simulink model "buckboostSMC2"  (R2024a)
settings: Solver=ode2  StartTime=0.0  StopTime=20  FixedStep=0.0001  RelTol=1e-3
InitFcn:
  | paramsTCST
values from neighbouring files (symbols this model uses):
  C = 2610*10^-6    (= 0.00261)    [SITLparameters.m]
  k1 = 0.022    [SITLparameters.m]
  k2 = 10    [SITLparameters.m]
  L = 2010*10^-6    (= 0.00201)    [SITLparameters.m]
  R = 25    [SITLparameters.m]
undefined symbols (not defined in the file or in its folder): gains, Lsig, Msig, params, Vd, x2d
settings Model: Creator=gerar  LastModifiedBy=rodol
settings ModelReferenceCC: EnableRefExpFcnMdlSchedulingChecks=on
settings RTWCC: GPUComputeCapability=3.5

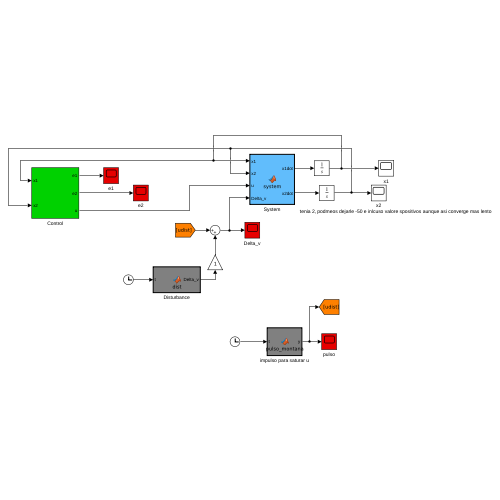
[thumbnail: Simulink's stored preview of the top-level diagram]
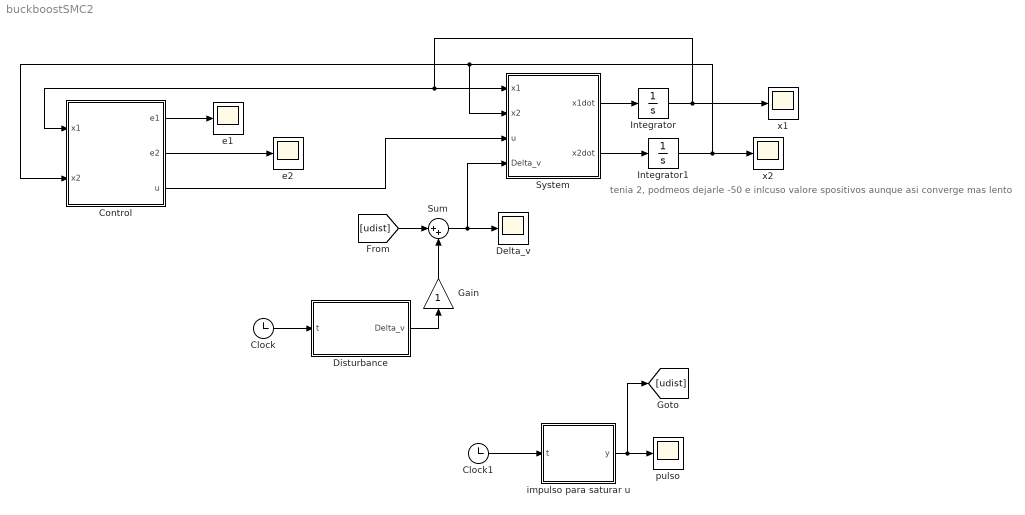
== system buckboostSMC2 ==
  note: tenia 2, podmeos dejarle -50 e inlcuso valore spositivos aunque asi converge mas lento
  Clock : Clock
  Clock1 : Clock
  Control : Subsystem
  Delta_v : Scope
  Disturbance : MATLAB Function  TreatAsAtomicUnit=on
  Gain : Gain
  Integrator : Integrator
  Integrator1 : Integrator  InitialCondition=-50
  Sum : Sum  Inputs=|++
  System : MATLAB Function  TreatAsAtomicUnit=on
  e1 : Scope
  e2 : Scope
  impulso para saturar u : MATLAB Function  TreatAsAtomicUnit=on
  pulso : Scope
  x1 : Scope
  x2 : Scope
  wires:
  System/1(x1dot) -> Integrator/1
  System/2(x2dot) -> Integrator1/1
  Integrator/1 -> x1/1, System/1(x1), Control/1(x1)
  Integrator1/1 -> x2/1, System/2(x2), Control/2(x2)
  Control/1(e1) -> e1/1
  Control/2(e2) -> e2/1
  Disturbance/1(Delta_v) -> Gain/1
  Clock/1 -> Disturbance/1(t)
  Control/3(u) -> System/3(u)
  Clock1/1 -> impulso para saturar u/1(t)
  impulso para saturar u/1(y) -> [udist], pulso/1
  Gain/1 -> Sum/2
  [udist] -> Sum/1
  Sum/1 -> System/4(Delta_v), Delta_v/1

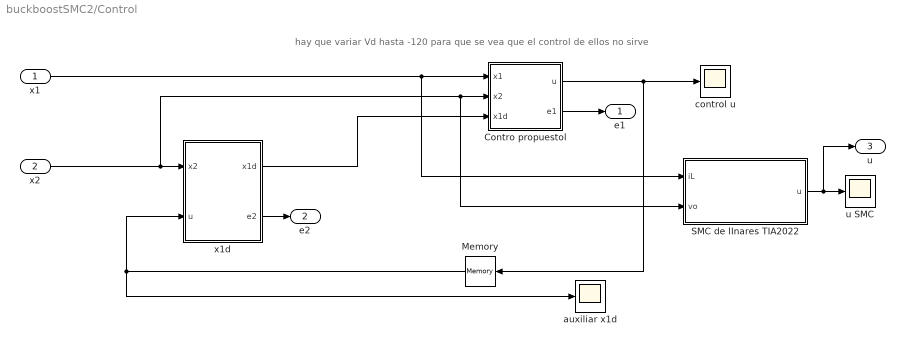
== system buckboostSMC2/Control ==
  note: hay que variar Vd hasta -120 para que se vea que el control de ellos no sirve
  x1 : Inport
  x2 : Inport  Port=2
  Contro propuestol : MATLAB Function  TreatAsAtomicUnit=on
  Memory : Memory
  SMC de lInares TIA2022 : MATLAB Function  TreatAsAtomicUnit=on
  auxiliar x1d : Scope
  control u : Scope
  u SMC : Scope
  x1d : MATLAB Function  TreatAsAtomicUnit=on
  e1 : Outport
  e2 : Outport  Port=2
  u : Outport  Port=3
  wires:
  x1d/1(x1d) -> Contro propuestol/3(x1d)
  x1/1 -> Contro propuestol/1(x1), SMC de lInares TIA2022/1(iL)
  x2/1 -> SMC de lInares TIA2022/2(vo), Contro propuestol/2(x2), x1d/1(x2)
  Memory/1 -> x1d/2(u), auxiliar x1d/1
  x1d/2(e2) -> e2/1
  Contro propuestol/2(e1) -> e1/1
  Contro propuestol/1(u) -> control u/1, Memory/1
  SMC de lInares TIA2022/1(u) -> u/1, u SMC/1

== matlab function buckboostSMC2/Control/Contro propuestol ==
  data: x1 input; u output; x2 input; x1d input; E parameter; R parameter; C parameter; L parameter; k1 parameter; k2 parameter; e1 output; Msig parameter; Lsig parameter
% function [u, e1] = control(x1, x2, x1d, x1d_dot, E, R, C, L, k1, k2)
% 
% %error
% e1 = x1 - x1d;
% 
% %control
% u = ( (  k1*L*15*(e1) + E  ) / ( x2 - E) ) + 1;



function [u, e1] = control(x1, x2, x1d, E, R, C, L, k1, k2, Msig, Lsig)
% CONTROL  Nonlinear control with semi-saturation sigma(·) from the paper
%
% Inputs:
%   x1, x2     - states (i_L, v_o)
%   x1d        - desired inductor current i_L^d
%   x1d_dot    - d/dt(i_L^d) (not used here, kept for interface completeness)
%   E, R, C, L - converter parameters
%   k1, k2     - control gains (k2 not used in this channel)
%   Lsig       - lower knee of semi-saturation σ(·) (default: 0)
%   Msig       - upper plateau of σ(·) (default: 0.95)
%
% Output:
%   u  - duty command after semi-saturation
%   e1 - current tracking error

    % defaults for sigma if not provided
    if nargin < 11 || isempty(Lsig), Lsig = 0;    end
    if nargin < 12 || isempty(Msig), Msig = 0.95; end   % ensure Msig < 1

    % error
    e1 = x1 - x1d;

    % ---------- Inner (unsaturated) control term ----------
    % NOTE: you provided this structure; we keep it as the inner command s.
    % Be careful with (x2 - E) near zero — sigma will keep u < Msig to avoid u=1.
    s = ( (k1*L*sign(e1)*sqrt(abs(e1)) + E ) / (x2 - E) ) + 1 ;

    % ---------- Semi-saturation σ(·) from the paper ----------
    % σ(s) = (1/c) * tanh(c*(s - Lsig)) + Lsig,   if s >= Lsig
    %         s                                  , otherwise
    % with c = pi/(2*(Msig - Lsig)) so that sup σ(s) < Msig < 1
    c = pi / (2 * (Msig - Lsig));

    if s >= Lsig
        u = (1/c) * tanh(c*(s - Lsig)) + Lsig;
    else
        u = s;
    end

    % (Opcional) seguridad numérica para forzar límites duros si lo prefieres:
    % u = min(u, Msig);

end

== matlab function buckboostSMC2/System ==
  data: x1 input; x2 input; u input; Delta_v input; x1dot output; x2dot output; E parameter; R parameter; C parameter; L parameter
function [x1dot, x2dot] = system(x1, x2, u, Delta_v, E, R, C, L)

%System
x1dot = (1-u)*(1/L)*x2 + u*(E/L);
x2dot = -(1-u)*(1/C)*x1 - (1/( (R + 0*R)*C ))*x2 + Delta_v;

== matlab function buckboostSMC2/Control/x1d ==
  data: x1d output; x2 input; u input; k2 parameter; x2d parameter; C parameter; R parameter; e2 output
function [x1d, e2] = des(x2, u, k2, x2d, C, R)

%error
e2 = x2 - x2d;

%Auxiliar control
x1d = C * ( ( k2 * sign(e2)*sqrt(abs(e2)) - (1/(R*C))*x2 ) / (1 - u) ); % normal

== matlab function buckboostSMC2/Disturbance ==
  data: t input; Delta_v output
function Delta_v = dist(t)

Delta_v = 2*sin(0.5*t);

== matlab function buckboostSMC2/Control/SMC de lInares TIA2022 ==
  data: iL input; u output; vo input; gains parameter; params parameter; Vd parameter
function u = tsmc_bb(iL, vo, gains, params, Vd)
% params: struct with E,R,L,C  (+ opcional Ts, fsw)
% gains : struct with c, lambda, epsu
% Vd    : referencia de voltaje (negativa en el buck-boost inversor)
% ip    : perturbación de corriente (puedes pasar 0 si no la usas)

E = params.E; R = params.R; L = params.L; C = params.C;
c = gains.c;  lam = gains.lambda;

% === 1) Equilibrios del paper (ec. 3) y referencia x1d ===
ubar  = Vd/(Vd - E);
iLbar = Vd*(Vd - E)/(R*E);
x1d   = 0.5*( L*iLbar^2 + C*(E - Vd)^2 );   % Hbar

% === 2) Coordenadas planas (paper ec. 6) ===
x1 = 0.5*( L*iL^2 + C*(E - vo)^2 );
x2 = E*iL + (vo/R)*(E - vo);

% === 3) Dinámica linealizada: x1dot = x2 ; x2dot = alpha + beta*u + d_ip
alpha = E*vo/L + (2*vo - E)*( vo/(R^2*C) + iL/(R*C) );   % expresión del paper (en iL,vo)
beta  = (E*(E - vo))/L + (iL/(R*C))*(E - 2*vo);    % expresión del paper (en iL,vo)

% === 4) Superficie deslizante y ley TSMC (paper ec. 13–14) ===
sigma = c*(x1 - x1d) + x2;
u = -( alpha + c*x2 + lam*sign(sigma) ) / beta;

% === 6) Salidas auxiliares para depuracion ===
%aux.ubar  = ubar;     % duty en equilibrio (feedforward opcional)
%aux.iLbar = iLbar;    % corriente en equilibrio
%aux.x1    = x1; aux.x2 = x2; aux.x1d = x1d;
%aux.alpha = alpha; aux.beta = beta; aux.sigma = sigma;
end

== matlab function buckboostSMC2/impulso para saturar u ==
  data: t input; y output
function y = pulso_montana(t)
% y = pulso_montana(t, t0, t1, A)
% Pulso "montaña" suave:
%   - y = 0 antes de t0 y después de t1
%   - Sube suave de 0 a 1 entre t0 y (t0+t1)/2
%   - Baja suave de 1 a 0 entre (t0+t1)/2 y t1
%   - Amplitud A (por defecto 1)
%
% Recomendado: 
t0 = 5; t1 = 5.5; A = 10;

    if nargin < 4, A = 10; end

    if t <= t0 || t >= t1
        y = 0;
        return;
    end

    tc = 0.5*(t0 + t1);  % centro del pulso

    if t <= tc
        % fase de subida (0 → 1) con smootherstep
        u = (t - t0) / (tc - t0);          % u en [0,1]
        s = u^3 * (u * (u*6 - 15) + 10);   % smootherstep
        y = A * s;
    else
        % fase de bajada (1 → 0)
        u = (t - tc) / (t1 - tc);          % u en [0,1]
        s = u^3 * (u * (u*6 - 15) + 10);
        y = A * (1 - s);
    end
end
